simulink model "Clique"  (R2022b)
settings: Solver=VariableStepAuto  StartTime=0.0  StopTime=10000.0  RelTol=1e-3
settings Model: Creator=marpe  LastModifiedBy=marpe

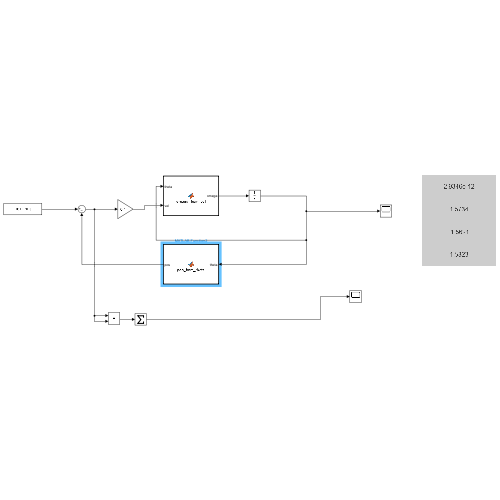
[thumbnail: Simulink's stored preview of the top-level diagram]
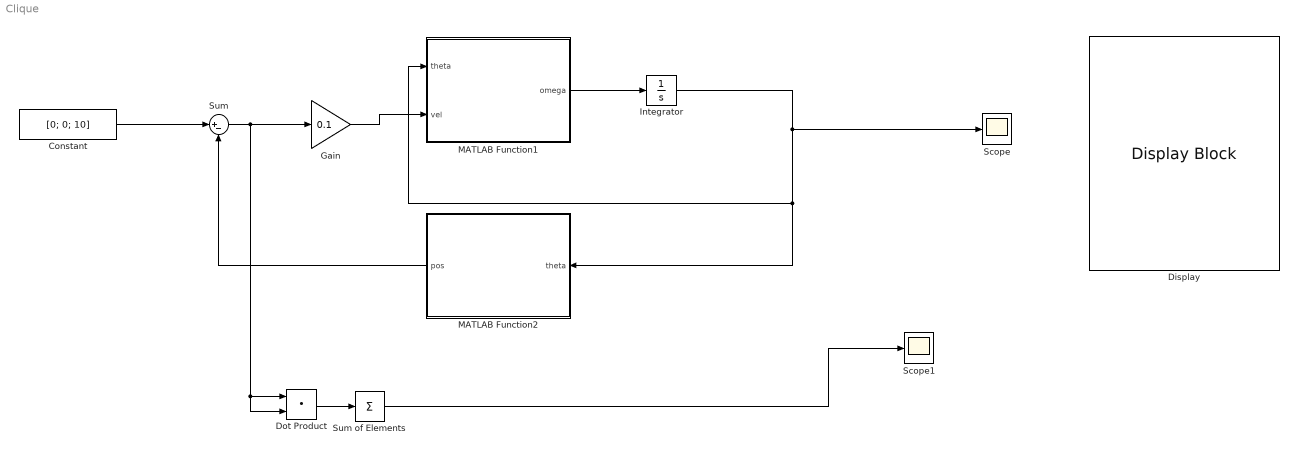
== system Clique ==
  Constant : Constant  Value=[0; 0; 10]  VectorParams1D=off
  Display : DisplayBlock  LabelPosition=Hide  Transparency=1
  Dot Product : DotProduct  OutDataTypeStr=Inherit: Inherit via internal rule
  Gain : Gain  Gain=0.1
  Integrator : Integrator  InitialCondition=[0; 0; 0; 0]
  MATLAB Function1 : MATLAB Function  TreatAsAtomicUnit=on
  MATLAB Function2 : MATLAB Function  TreatAsAtomicUnit=on
  Scope : Scope
  Scope1 : Scope
  Sum : Sum  Inputs=|+-
  Sum of Elements : Sum  Inputs=+
  wires:
  MATLAB Function2/1(pos) -> Sum/2
  Sum/1 -> Dot Product/2, Dot Product/1, Gain/1
  Gain/1 -> MATLAB Function1/2(vel)
  MATLAB Function1/1(omega) -> Integrator/1
  Integrator/1 -> Scope/1, MATLAB Function2/1(theta), MATLAB Function1/1(theta)
  Dot Product/1 -> Sum of Elements/1
  Sum of Elements/1 -> Scope1/1
  Constant/1 -> Sum/1

== matlab function Clique/MATLAB Function2 ==
  data: pos output; theta input
function pos = pos_from_theta(theta)
    PE_eval = @(th1,th2,th3,th4)[cos(th1).*cos(th2).*(5.9e+1./5.0)+cos(th4).*(cos(th1).*cos(th2).*sin(th3+pi./2.0)+cos(th1).*cos(th3+pi./2.0).*sin(th2)).*(9.4e+1./5.0)-sin(th4).*(cos(th1).*sin(th2).*sin(th3+pi./2.0)-cos(th1).*cos(th2).*cos(th3+pi./2.0)).*(9.4e+1./5.0)-cos(th1).*sin(th2).*sin(th3+pi./2.0).*(2.5e+1./2.0)+cos(th1).*cos(th2).*cos(th3+pi./2.0).*(2.5e+1./2.0);cos(th2).*sin(th1).*(5.9e+1./5.0)+cos(th4).*(cos(th2).*sin(th1).*sin(th3+pi./2.0)+cos(th3+pi./2.0).*sin(th1).*sin(th2)).*(9.4e+1./5.0)+sin(th4).*(cos(th2).*cos(th3+pi./2.0).*sin(th1)-sin(th1).*sin(th2).*sin(th3+pi./2.0)).*(9.4e+1./5.0)+cos(th2).*cos(th3+pi./2.0).*sin(th1).*(2.5e+1./2.0)-sin(th1).*sin(th2).*sin(th3+pi./2.0).*(2.5e+1./2.0);sin(th2).*(5.9e+1./5.0)+sin(th4).*(cos(th2).*sin(th3+pi./2.0)+cos(th3+pi./2.0).*sin(th2)).*(9.4e+1./5.0)+cos(th2).*sin(th3+pi./2.0).*(2.5e+1./2.0)+cos(th3+pi./2.0).*sin(th2).*(2.5e+1./2.0)-cos(th4).*(cos(th2).*cos(th3+pi./2.0)-sin(th2).*sin(th3+pi./2.0)).*(9.4e+1./5.0)+7.0];
    pos = PE_eval(theta(1, 1), theta(2, 1), theta(3, 1), theta(4, 1));

== matlab function Clique/MATLAB Function1 ==
  data: omega output; theta input; vel input
function omega = omega_from_vel(theta, vel)

    JPE_eval = @(th1,th2,th3,th4)reshape([cos(th2).*sin(th1).*(-5.9e+1./5.0)-cos(th4).*(cos(th2).*sin(th1).*sin(th3+pi./2.0)+cos(th3+pi./2.0).*sin(th1).*sin(th2)).*(9.4e+1./5.0)-sin(th4).*(cos(th2).*cos(th3+pi./2.0).*sin(th1)-sin(th1).*sin(th2).*sin(th3+pi./2.0)).*(9.4e+1./5.0)-cos(th2).*cos(th3+pi./2.0).*sin(th1).*(2.5e+1./2.0)+sin(th1).*sin(th2).*sin(th3+pi./2.0).*(2.5e+1./2.0),cos(th1).*cos(th2).*(5.9e+1./5.0)+cos(th4).*(cos(th1).*cos(th2).*sin(th3+pi./2.0)+cos(th1).*cos(th3+pi./2.0).*sin(th2)).*(9.4e+1./5.0)-sin(th4).*(cos(th1).*sin(th2).*sin(th3+pi./2.0)-cos(th1).*cos(th2).*cos(th3+pi./2.0)).*(9.4e+1./5.0)-cos(th1).*sin(th2).*sin(th3+pi./2.0).*(2.5e+1./2.0)+cos(th1).*cos(th2).*cos(th3+pi./2.0).*(2.5e+1./2.0),0.0,cos(th1).*sin(th2).*(-5.9e+1./5.0)-cos(th4).*(cos(th1).*sin(th2).*sin(th3+pi./2.0)-cos(th1).*cos(th2).*cos(th3+pi./2.0)).*(9.4e+1./5.0)-sin(th4).*(cos(th1).*cos(th2).*sin(th3+pi./2.0)+cos(th1).*cos(th3+pi./2.0).*sin(th2)).*(9.4e+1./5.0)-cos(th1).*cos(th2).*sin(th3+pi./2.0).*(2.5e+1./2.0)-cos(th1).*cos(th3+pi./2.0).*sin(th2).*(2.5e+1./2.0),sin(th1).*sin(th2).*(-5.9e+1./5.0)+cos(th4).*(cos(th2).*cos(th3+pi./2.0).*sin(th1)-sin(th1).*sin(th2).*sin(th3+pi./2.0)).*(9.4e+1./5.0)-sin(th4).*(cos(th2).*sin(th1).*sin(th3+pi./2.0)+cos(th3+pi./2.0).*sin(th1).*sin(th2)).*(9.4e+1./5.0)-cos(th2).*sin(th1).*sin(th3+pi./2.0).*(2.5e+1./2.0)-cos(th3+pi./2.0).*sin(th1).*sin(th2).*(2.5e+1./2.0),cos(th2).*(5.9e+1./5.0)+sin(th4).*(cos(th2).*cos(th3+pi./2.0)-sin(th2).*sin(th3+pi./2.0)).*(9.4e+1./5.0)+cos(th2).*cos(th3+pi./2.0).*(2.5e+1./2.0)-sin(th2).*sin(th3+pi./2.0).*(2.5e+1./2.0)+cos(th4).*(cos(th2).*sin(th3+pi./2.0)+cos(th3+pi./2.0).*sin(th2)).*(9.4e+1./5.0),cos(th4).*(cos(th1).*sin(th2).*sin(th3+pi./2.0)-cos(th1).*cos(th2).*cos(th3+pi./2.0)).*(-9.4e+1./5.0)-sin(th4).*(cos(th1).*cos(th2).*sin(th3+pi./2.0)+cos(th1).*cos(th3+pi./2.0).*sin(th2)).*(9.4e+1./5.0)-cos(th1).*cos(th2).*sin(th3+pi./2.0).*(2.5e+1./2.0)-cos(th1).*cos(th3+pi./2.0).*sin(th2).*(2.5e+1./2.0),cos(th4).*(cos(th2).*cos(th3+pi./2.0).*sin(th1)-sin(th1).*sin(th2).*sin(th3+pi./2.0)).*(9.4e+1./5.0)-sin(th4).*(cos(th2).*sin(th1).*sin(th3+pi./2.0)+cos(th3+pi./2.0).*sin(th1).*sin(th2)).*(9.4e+1./5.0)-cos(th2).*sin(th1).*sin(th3+pi./2.0).*(2.5e+1./2.0)-cos(th3+pi./2.0).*sin(th1).*sin(th2).*(2.5e+1./2.0),sin(th4).*(cos(th2).*cos(th3+pi./2.0)-sin(th2).*sin(th3+pi./2.0)).*(9.4e+1./5.0)+cos(th2).*cos(th3+pi./2.0).*(2.5e+1./2.0)-sin(th2).*sin(th3+pi./2.0).*(2.5e+1./2.0)+cos(th4).*(cos(th2).*sin(th3+pi./2.0)+cos(th3+pi./2.0).*sin(th2)).*(9.4e+1./5.0),cos(th4).*(cos(th1).*sin(th2).*sin(th3+pi./2.0)-cos(th1).*cos(th2).*cos(th3+pi./2.0)).*(-9.4e+1./5.0)-sin(th4).*(cos(th1).*cos(th2).*sin(th3+pi./2.0)+cos(th1).*cos(th3+pi./2.0).*sin(th2)).*(9.4e+1./5.0),cos(th4).*(cos(th2).*cos(th3+pi./2.0).*sin(th1)-sin(th1).*sin(th2).*sin(th3+pi./2.0)).*(9.4e+1./5.0)-sin(th4).*(cos(th2).*sin(th1).*sin(th3+pi./2.0)+cos(th3+pi./2.0).*sin(th1).*sin(th2)).*(9.4e+1./5.0),sin(th4).*(cos(th2).*cos(th3+pi./2.0)-sin(th2).*sin(th3+pi./2.0)).*(9.4e+1./5.0)+cos(th4).*(cos(th2).*sin(th3+pi./2.0)+cos(th3+pi./2.0).*sin(th2)).*(9.4e+1./5.0)],[3,4]);
    J = JPE_eval(theta(1, 1), theta(2, 1), theta(3, 1), theta(4, 1));
    invJ = pinv(J);
    omega = invJ*vel;
